simulink model "pos_8mot"  (R2021a)
settings: Solver=FixedStepDiscrete  StartTime=0.0  StopTime=inf  FixedStep=0.001  RelTol=1e-3  EnableMultiTasking=on
InitFcn:
  | load("rho_CommandCalib.mat");
  | run("importCmd.m")
model workspace (MAT data in the model file):
  positionCmd = [145.742 145.741 145.741 145.74 145.74 145.739 145.738 145.738 145.737 145.737 145.736 145.735 ... (560000 elements, 70000x8)]
  tempsTraj = [25 25 20]
values from neighbouring files (symbols this model uses):
  rho_CommandCalib = [325.033 325.033 325.033 325.033 325.033 325.033 325.033 325.033 325.033 325.033 325.033 325.033 ... (80000 elements, 10000x8)]    [rho_CommandCalib.mat]
undefined symbols (not defined in the file or in its folder): rho_CommandCircXY, rho_CommandCroixTilt, rho_CommandCroixXY, rho_CommandInclinaison, rho_CommandInclinaisonInterieure, rho_CommandPickAndPlace, rho_CommandPickAndPlaceTilt, rho_CommandPickAndPlaceVertical, rho_CommandPickAndPlaceX, rho_CommandSinusZ, rho_CommandSinusZ_decentree, rho_CommandTwist
libraries: xpcethercatlib x64, slrealtimeethercatlib x36, commutil2 x19, slrealtimeobsoletelib x7
(part 3 of 3)

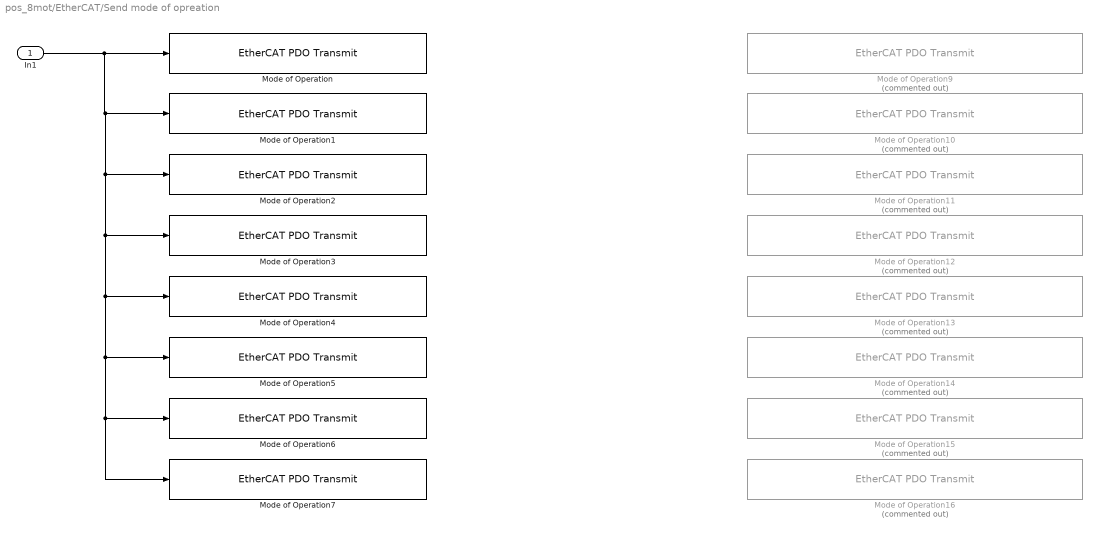
== system pos_8mot/EtherCAT/Send mode of opreation ==
  In1 : Inport
  Mode of Operation : xpcethercatlib/EtherCAT PDO Transmit   Priority=3  sig_name=Drive 1 (C1150-DS-XC-0S).Cylic Position Mode.Mode of Operation  sig_offset=744  sig_type=int8  type_size=8  sig_dim=1  device_id=0  sample_time=0.001000
      settings: SourceProductBaseCode=XP
  Mode of Operation1 : xpcethercatlib/EtherCAT PDO Transmit   Priority=3  sig_name=Drive 2 (C1150-DS-XC-0S).Cylic Position Mode.Mode of Operation  sig_offset=920  sig_type=int8  type_size=8  sig_dim=1  device_id=0  sample_time=0.001000
      settings: SourceProductBaseCode=XP
  Mode of Operation10 : xpcethercatlib/EtherCAT PDO Transmit   Priority=3  Commented=on  sig_name=Drive 2 (C1150-DS-XC-0S).Cylic Position Velocity Mode.Mode of Operation  sig_offset=936  sig_type=int8  type_size=8  sig_dim=1  device_id=0  sample_time=0.001000
      settings: SourceProductBaseCode=XP
  Mode of Operation11 : xpcethercatlib/EtherCAT PDO Transmit   Priority=3  Commented=on  sig_name=Drive 3 (C1150-DS-XC-0S).Cylic Position Velocity Mode.Mode of Operation  sig_offset=1080  sig_type=int8  type_size=8  sig_dim=1  device_id=0  sample_time=0.001000
      settings: SourceProductBaseCode=XP
  Mode of Operation12 : xpcethercatlib/EtherCAT PDO Transmit   Priority=3  Commented=on  sig_name=Drive 4 (C1150-DS-XC-0S).Cylic Position Velocity Mode.Mode of Operation  sig_offset=1224  sig_type=int8  type_size=8  sig_dim=1  device_id=0  sample_time=0.001000
      settings: SourceProductBaseCode=XP
  Mode of Operation13 : xpcethercatlib/EtherCAT PDO Transmit   Priority=3  Commented=on  sig_name=Drive 5 (C1150-DS-XC-0S).Cylic Position Velocity Mode.Mode of Operation  sig_offset=1368  sig_type=int8  type_size=8  sig_dim=1  device_id=0  sample_time=0.001000
      settings: SourceProductBaseCode=XP
  Mode of Operation14 : xpcethercatlib/EtherCAT PDO Transmit   Priority=3  Commented=on  sig_name=Drive 6 (C1150-DS-XC-0S).Cylic Position Velocity Mode.Mode of Operation  sig_offset=1512  sig_type=int8  type_size=8  sig_dim=1  device_id=0  sample_time=0.001000
      settings: SourceProductBaseCode=XP
  Mode of Operation15 : xpcethercatlib/EtherCAT PDO Transmit   Priority=3  Commented=on  sig_name=Drive 7 (C1150-DS-XC-0S).Cylic Position Velocity Mode.Mode of Operation  sig_offset=1656  sig_type=int8  type_size=8  sig_dim=1  device_id=0  sample_time=0.001000
      settings: SourceProductBaseCode=XP
  Mode of Operation16 : xpcethercatlib/EtherCAT PDO Transmit   Priority=3  Commented=on  sig_name=Drive 8 (C1150-DS-XC-0S).Cylic Position Velocity Mode.Mode of Operation  sig_offset=1800  sig_type=int8  type_size=8  sig_dim=1  device_id=0  sample_time=0.001000
      settings: SourceProductBaseCode=XP
  Mode of Operation2 : xpcethercatlib/EtherCAT PDO Transmit   Priority=3  sig_name=Drive 3 (C1150-DS-XC-0S).Cylic Position Mode.Mode of Operation  sig_offset=1080  sig_type=int8  type_size=8  sig_dim=1  device_id=0  sample_time=0.001000
      settings: SourceProductBaseCode=XP
  Mode of Operation3 : xpcethercatlib/EtherCAT PDO Transmit   Priority=3  sig_name=Drive 4 (C1150-DS-XC-0S).Cylic Position Mode.Mode of Operation  sig_offset=1240  sig_type=int8  type_size=8  sig_dim=1  device_id=0  sample_time=0.001000
      settings: SourceProductBaseCode=XP
  Mode of Operation4 : xpcethercatlib/EtherCAT PDO Transmit   Priority=3  sig_name=Drive 5 (C1150-DS-XC-0S).Cylic Position Mode.Mode of Operation  sig_offset=1400  sig_type=int8  type_size=8  sig_dim=1  device_id=0  sample_time=0.001000
      settings: SourceProductBaseCode=XP
  Mode of Operation5 : xpcethercatlib/EtherCAT PDO Transmit   Priority=3  sig_name=Drive 6 (C1150-DS-XC-0S).Cylic Position Mode.Mode of Operation  sig_offset=1560  sig_type=int8  type_size=8  sig_dim=1  device_id=0  sample_time=0.001000
      settings: SourceProductBaseCode=XP
  Mode of Operation6 : xpcethercatlib/EtherCAT PDO Transmit   Priority=3  sig_name=Drive 7 (C1150-DS-XC-0S).Cylic Position Mode.Mode of Operation  sig_offset=1720  sig_type=int8  type_size=8  sig_dim=1  device_id=0  sample_time=0.001000
      settings: SourceProductBaseCode=XP
  Mode of Operation7 : xpcethercatlib/EtherCAT PDO Transmit   Priority=3  sig_name=Drive 8 (C1150-DS-XC-0S).Cylic Position Mode.Mode of Operation  sig_offset=1880  sig_type=int8  type_size=8  sig_dim=1  device_id=0  sample_time=0.001000
      settings: SourceProductBaseCode=XP
  Mode of Operation9 : xpcethercatlib/EtherCAT PDO Transmit   Priority=3  Commented=on  sig_name=Drive 1 (C1150-DS-XC-0S).Cylic Position Velocity Mode.Mode of Operation  sig_offset=776  sig_type=int8  type_size=8  sig_dim=1  device_id=0  sample_time=0.001000
      settings: SourceProductBaseCode=XP
  wires:
  In1/1 -> Mode of Operation7/1, Mode of Operation6/1, Mode of Operation5/1, Mode of Operation4/1, Mode of Operation3/1, Mode of Operation2/1, Mode of Operation1/1, Mode of Operation/1

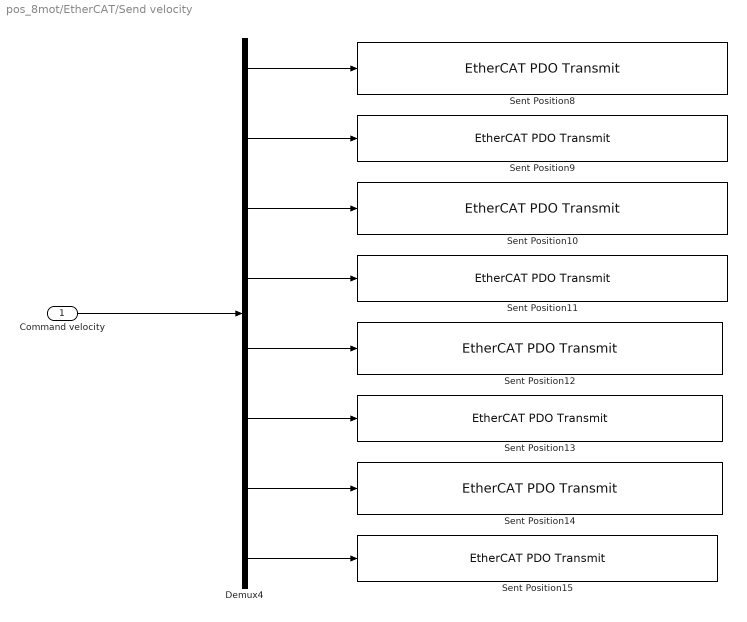
== system pos_8mot/EtherCAT/Send velocity ==
  Command velocity : Inport
  Demux4 : Demux  Outputs=8
  Sent Position10 : xpcethercatlib/EtherCAT PDO Transmit   Priority=3  sig_name=Drive 3 (C1150-DS-XC-0S).Cylic Position Velocity Mode.Target velocity  sig_offset=1048  sig_type=int32  type_size=32  sig_dim=1  device_id=0  sample_time=0.001000
      settings: SourceProductBaseCode=XP
  Sent Position11 : xpcethercatlib/EtherCAT PDO Transmit   Priority=3  sig_name=Drive 4 (C1150-DS-XC-0S).Cylic Position Velocity Mode.Target velocity  sig_offset=1192  sig_type=int32  type_size=32  sig_dim=1  device_id=0  sample_time=0.001000
      settings: SourceProductBaseCode=XP
  Sent Position12 : xpcethercatlib/EtherCAT PDO Transmit   Priority=3  sig_name=Drive 5 (C1150-DS-XC-0S).Cylic Position Velocity Mode.Target velocity  sig_offset=1336  sig_type=int32  type_size=32  sig_dim=1  device_id=0  sample_time=0.001000
      settings: SourceProductBaseCode=XP
  Sent Position13 : xpcethercatlib/EtherCAT PDO Transmit   Priority=3  sig_name=Drive 6 (C1150-DS-XC-0S).Cylic Position Velocity Mode.Target velocity  sig_offset=1480  sig_type=int32  type_size=32  sig_dim=1  device_id=0  sample_time=0.001000
      settings: SourceProductBaseCode=XP
  Sent Position14 : xpcethercatlib/EtherCAT PDO Transmit   Priority=3  sig_name=Drive 7 (C1150-DS-XC-0S).Cylic Position Velocity Mode.Target velocity  sig_offset=1624  sig_type=int32  type_size=32  sig_dim=1  device_id=0  sample_time=0.001000
      settings: SourceProductBaseCode=XP
  Sent Position15 : xpcethercatlib/EtherCAT PDO Transmit   Priority=3  sig_name=Drive 8 (C1150-DS-XC-0S).Cylic Position Velocity Mode.Target velocity  sig_offset=1768  sig_type=int32  type_size=32  sig_dim=1  device_id=0  sample_time=0.001000
      settings: SourceProductBaseCode=XP
  Sent Position8 : xpcethercatlib/EtherCAT PDO Transmit   Priority=3  sig_name=Drive 1 (C1150-DS-XC-0S).Cylic Position Velocity Mode.Target velocity  sig_offset=744  sig_type=int32  type_size=32  sig_dim=1  device_id=0  sample_time=0.001000
      settings: SourceProductBaseCode=XP
  Sent Position9 : xpcethercatlib/EtherCAT PDO Transmit   Priority=3  sig_name=Drive 2 (C1150-DS-XC-0S).Cylic Position Velocity Mode.Target velocity  sig_offset=904  sig_type=int32  type_size=32  sig_dim=1  device_id=0  sample_time=0.001000
      settings: SourceProductBaseCode=XP
  wires:
  Demux4/1 -> Sent Position8/1
  Demux4/4 -> Sent Position11/1
  Demux4/7 -> Sent Position14/1
  Demux4/2 -> Sent Position9/1
  Demux4/8 -> Sent Position15/1
  Demux4/6 -> Sent Position13/1
  Demux4/5 -> Sent Position12/1
  Demux4/3 -> Sent Position10/1
  Command velocity/1 -> Demux4/1

== matlab function pos_8mot/EtherCAT/MATLAB Function8 ==
  data: y output; u input
function y = clignote(u)


frequence_clignotement = 1; % 1 fois par seconde
frequence_solver = 1000; % Hz

mode = u(1);

reset_counter = u(2);

persistent etat;
if isempty(etat)
    etat = 0; % Éteinte
end

persistent i;
if isempty(i)
    i = 1;
elseif reset_counter == 1
    i = 1;
    etat = 0;
    mode = 0;
end



if mode == 0
    etat = 0; % Éteinte
    
elseif mode == 1
      
    etat = 1; % Allumée
    
elseif mode == 0.5 % Clignote

    if i > frequence_solver/frequence_clignotement % Fréquence de clignotement de 1 Hz
        i = 0;
        % Changement d'état
        if etat == 1
            etat = 0;
        else
            etat = 1;
        end
    end
    
else
    etat = 0; % Éteinte
end
    

i = i + 1;

if i > 60*60*24*frequence_solver % Number of increment in 1 day at frequence_solver Hz
    
    i = 1;
    
end


y = etat;

== matlab function pos_8mot/EtherCAT/MATLAB Function9 ==
  data: trajectorySelector input; target output size=[1 8]; pause input; stopAtEnd input; isCompleted output; waitForActivation input; position_from_gabarit_to_standby input; positionCmd parameter; tempsTraj parameter
function [target,isCompleted] = trajectoryManager(trajectorySelector,pause,stopAtEnd,waitForActivation,position_from_gabarit_to_standby, positionCmd, tempsTraj)

	% Constants declaration
	persistent index %index of the table trajectory
	if isempty(index)
		index = 1;
	end
	
	
	persistent flag_stopAtEnd % To stop the endless loop trajectory at the end of current trajectory
    if isempty(flag_stopAtEnd)
		flag_stopAtEnd = 0;
    end
    
    persistent numTraj
    persistent currentTime
    persistent currentIndex
    if isempty(numTraj)
        numTraj = 1;
        currentTime = tempsTraj(numTraj); %Init temps de la première trajectoire
        currentIndex = 2;
    end
	
	
	persistent pos %position of the actuator of the robot
	if isempty(pos) % Les valeurs de calibrations
		pos = [325, 323.80, 325, 325, 293.60, 293.25, 316.76, 318.94]; % 1x8 vector TO CHANGE WITH REAL CALIBRATION VALUES
	%     pos = 325; % For tests with only 1 actuator
	
	end
	
	
	
	trajectory_completed = 0; % Output variable to know if we've reach the end of a trajectory
	
	% Trajectory management
	
	
	if ~waitForActivation % If we are currently in a moving procedure
		
	
		if trajectorySelector == 1 % Trajectory from gabarit to standby
	
		   if index == length(position_from_gabarit_to_standby)
	
			   trajectory_completed = 1;
			   index = 1;
			   pos =  position_from_gabarit_to_standby(end,:);
		   else
			   if ~pause
				   index = index + 1;
			   end
			   
			   % Because of unit delay to notify that the trajectory is
			   % completed, the last command sent to actuators won't be when
			   % index = length(trajectory), but index = 1 because of the
			   % re-initialization of index when index = length(trajectory). To
			   % prevent this discontinuity in the position command, we must
			   % ensure that if the present position of actuators corresponds
			   % to the last position of trajectory vector, then we hold that
			   % position. Not optimal, but functionnal.
			   if pos ~= position_from_gabarit_to_standby(end,:)
				   
				   pos =  position_from_gabarit_to_standby(index,:);
			   else
				   
				   pos = position_from_gabarit_to_standby(end,:);
			   end
		   end
	
	
	
		elseif trajectorySelector == 2 % Trajectory from standby to gabarit
	
		   if index == length(position_from_gabarit_to_standby)
	
			   trajectory_completed = 1;
			   index = 1;
			   pos =  position_from_gabarit_to_standby(1,:);
		   else
			   if ~pause
				   index = index + 1;
			   end
			   
			   if pos ~= position_from_gabarit_to_standby(1,:)
				   
				   % Reading Trajectory_from_gabarit_to_standby backway
				   pos =  position_from_gabarit_to_standby(length(position_from_gabarit_to_standby)-index+1,:);
			   else
				   pos = position_from_gabarit_to_standby(1,:);
			   end  
		   end
	
	
	
	
	
	
	
	
		elseif trajectorySelector == 3 % Endless loop demo trajectory

			if currentIndex == currentTime * 1000
				currentIndex = 0;
                if numTraj == length(tempsTraj)     % After completing the last demo trajectory, we start again the neverending loop
                    index = 1;
                    pos =  positionCmd(end,:);
                    numTraj = 1;
                    currentIndex = 1;
                else
                    numTraj = numTraj + 1;
                end
                currentTime = tempsTraj(numTraj);
                
                if stopAtEnd
					trajectory_completed = 1;
                    index = 1;
                    numTraj = 1;
                    currentTime = tempsTraj(numTraj);
                    currentIndex = 1;
                end
			else
				if ~pause
					index = index + 1;
                    currentIndex = currentIndex + 1;
				end
				pos =  positionCmd(index,:);
			end
		else
			
			% Do nothing, stay in the current configuration
	
		end
	
	else
		
		% Holds the current configuration with persistent variable pos
		
	end
	
	
	target = pos;
	isCompleted = trajectory_completed;
	
	end

== matlab function pos_8mot/EtherCAT/Activation1/controlWord Generator ==
  data: mode output; controlword output; action input; stop input
function [mode, controlword] = fcn(action, stop)
%#codegen

persistent power
if isempty(power)
    power = 0;
end
persistent homing
if isempty(homing)
    homing = 0;
end

controlword = [0;0;1;0;0;0];
mode = 8;
if stop == 0
    if action==1 %arret
        controlword = [0;0;1;0;0;0];
        power = 0;
    elseif action==2 %homing de la position du moteur
        mode = 6;
        if power==0
            controlword = [0;1;1;1;0;0];
            power = 1;
        elseif power==1 && homing==0
            controlword = [1;1;1;1;0;0];
            homing = 1;
        elseif homing==1
            controlword = [1;1;1;1;1;0];
        end
    elseif action==3 %active la drive
        if power==0
            controlword = [0;1;1;1;0;0];
            power = 1;
        else
            controlword = [1;1;1;1;0;0];
        end
    elseif action==4 %reset fautes
        controlword = [0;1;1;1;0;1];
        power = 0;
        homing = 0;
    end
end

== matlab function pos_8mot/EtherCAT/MATLAB Function ==
  data: y output; u input
function y = clignote(u)


mode = u(1);

frequence_clignotement = 1; % 1 fois par seconde
frequence_solver = 1000; % Hz



persistent i;
if isempty(i)
    i = 1;
% elseif resetCounter == 1 % Changement d'état
%     i = 1;
end

persistent etat;
if isempty(etat)
    etat = 0; % Éteinte
end

if mode == 0
    etat = 0; % Éteinte
    
elseif mode == 1
    etat = 1; % Allumée
    
elseif mode == 0.5 % Clignote

    if i > frequence_solver/frequence_clignotement % Fréquence de clignotement de 1 Hz
        i = 0;
        % Changement d'état
        if etat == 1
            etat = 0;
        else
            etat = 1;
        end
    end
    
else
    etat = 0; % Éteinte
end
    

i = i + 1;

if i > 60*60*24*frequence_solver % Number of increment in 1 day at frequence_solver Hz
    
    i = 1;
    
end


y = etat;

== matlab function pos_8mot/EtherCAT/MATLAB Function1 ==
  data: buttonState input; isPressed output
% This function determines if a button has been pressed, in other words, if
% a rising edge followed by a falling edge has been detected.

% buttonState [0,1]

function isPressed = buttonPressed(buttonState)


buttonState = double(buttonState);

% Variable declaration

frequence_solver = 1000; % Hz

minimumPulseWidth = 0.1*frequence_solver; % Minimum allowable pulse width to accept pushed button, sec*Hz

isPressed = 0;

persistent i;
if isempty(i)
    i = 1;
end

persistent i_risingEdge;
if isempty(i_risingEdge)
    i_risingEdge = 1;
end

persistent i_fallingEdge;
if isempty(i_fallingEdge)
    i_fallingEdge = 1;
end


persistent pastState;
if isempty(pastState)
    pastState = 0;
end

persistent presentState;
if isempty(presentState)
    presentState = 0;
else
    presentState = buttonState;
end






% Rising edge detection
if pastState == 0 && presentState == 1

    i_risingEdge = i;

end

% Falling edge detection
if pastState == 1 && presentState == 0

    i_fallingEdge = i;
    
    if i_fallingEdge - i_risingEdge > minimumPulseWidth % To avoid button flickering
        
        isPressed = 1;
        
    else
        
        isPressed = 0;
        
    end

end




i = i + 1;

if i > 60*60*24*frequence_solver % Number of increments in 1 day at frequence_solver Hz
    
    i = 1;
    
end


pastState = presentState;


end

== matlab function pos_8mot/EtherCAT/MATLAB Function2 ==
  data: input input; new_state output; state input; output output
function [new_state,output] = fcn(input,state)

STATE_INIT = 0; 
STATE_WAIT_ECAT = 1; % wait ecat 8
STATE_WAIT_GABARIT_BUTTON = 2; 
STATE_CALIBRATION = 3; % set offsets for actuators
STATE_WAIT_INIT_MOVE_BUTTON = 4; 
STATE_DO_INITIAL_MOVE = 5; 
STATE_WAIT_NEW_TRAJ_BUTTON = 6; 
STATE_DO_REFERENCE_MOVE = 7; 
STATE_DO_REFERENCE_MOVE_LAST = 8; 
STATE_END = 100; 

ecat_state = input(1); 
button_1 = input(2); 
button_2 = input(3); 
button_3 = input(4); 
init_traj_end = input(5); 
ref_traj_end = input(6); 

new_state = -1; 

if state == STATE_INIT
    new_state = STATE_WAIT_ECAT; 
elseif state == STATE_WAIT_ECAT
    if ecat_state == 8
        new_state = STATE_WAIT_GABARIT_BUTTON; 
    else
        new_state = STATE_WAIT_ECAT; 
    end
elseif state == STATE_WAIT_GABARIT_BUTTON
    if button_1 == 1
        new_state = STATE_CALIBRATION; 
    else
        new_state = STATE_WAIT_GABARIT_BUTTON; 
    end
elseif state == STATE_CALIBRATION
    new_state = STATE_WAIT_INIT_MOVE_BUTTON; 
elseif state == STATE_WAIT_INIT_MOVE_BUTTON
    if button_2 == 1
        new_state = STATE_DO_INITIAL_MOVE; 
    else
        new_state = STATE_WAIT_INIT_MOVE_BUTTON; 
    end
elseif state == STATE_DO_INITIAL_MOVE
    if init_traj_end == 1
        new_state = STATE_WAIT_NEW_TRAJ_BUTTON; 
    else
        new_state = STATE_DO_INITIAL_MOVE; 
    end
elseif state == STATE_WAIT_NEW_TRAJ_BUTTON
    if button_3 == 1
        new_state = STATE_DO_REFERENCE_MOVE; 
    else
        new_state = STATE_WAIT_NEW_TRAJ_BUTTON; 
    end
elseif state == STATE_DO_REFERENCE_MOVE
    if button_1 == 1
        new_state = STATE_DO_REFERENCE_MOVE_LAST; 
    else
        new_state = STATE_DO_REFERENCE_MOVE; 
    end
elseif state == STATE_DO_REFERENCE_MOVE_LAST
    if ref_traj_end == 1
        new_state = STATE_END; 
    else
        new_state = STATE_DO_REFERENCE_MOVE_LAST; 
    end
end











output = 0; 

if state == STATE_INIT
    output = 0; 
elseif state == STATE_WAIT_ECAT
    output = 0; 
elseif state == STATE_WAIT_GABARIT_BUTTON
    output = 0; 
elseif state == STATE_CALIBRATION
    output = 0; 
elseif state == STATE_WAIT_INIT_MOVE_BUTTON
    output = 0; 
elseif state == STATE_DO_INITIAL_MOVE
    output = 1; 
end



% new_states = fcn(inputs,states); 

end

== matlab function pos_8mot/EtherCAT/MATLAB Function3 ==
  data: buttonState input; isPressed output
% This function determines if a button has been pressed, in other words, if
% a rising edge followed by a falling edge has been detected.

% buttonState [0,1]

function isPressed = buttonPressed(buttonState)


buttonState = double(buttonState);

% Variable declaration

frequence_solver = 1000; % Hz

minimumPulseWidth = 0.1*frequence_solver; % Minimum allowable pulse width to accept pushed button, sec*Hz

isPressed = 0;

persistent i;
if isempty(i)
    i = 1;
end

persistent i_risingEdge;
if isempty(i_risingEdge)
    i_risingEdge = 1;
end

persistent i_fallingEdge;
if isempty(i_fallingEdge)
    i_fallingEdge = 1;
end


persistent pastState;
if isempty(pastState)
    pastState = 0;
end

persistent presentState;
if isempty(presentState)
    presentState = 0;
else
    presentState = buttonState;
end






% Rising edge detection
if pastState == 0 && presentState == 1

    i_risingEdge = i;

end

% Falling edge detection
if pastState == 1 && presentState == 0

    i_fallingEdge = i;
    
    if i_fallingEdge - i_risingEdge > minimumPulseWidth % To avoid button flickering
        
        isPressed = 1;
        
    else
        
        isPressed = 0;
        
    end

end




i = i + 1;

if i > 60*60*24*frequence_solver % Number of increment in 1 day at frequence_solver Hz
    
    i = 1;
    
end


pastState = presentState;

% isPressed = presentState;

end

== matlab function pos_8mot/EtherCAT/MATLAB Function4 ==
  data: buttonState input; isPressed output
% This function determines if a button has been pressed, in other words, if
% a rising edge followed by a falling edge has been detected.

% buttonState [0,1]

function isPressed = buttonPressed(buttonState)


buttonState = double(buttonState);

% Variable declaration

frequence_solver = 1000; % Hz

minimumPulseWidth = 0.1*frequence_solver; % Minimum allowable pulse width to accept pushed button, sec*Hz

isPressed = 0;

persistent i;
if isempty(i)
    i = 1;
end

persistent i_risingEdge;
if isempty(i_risingEdge)
    i_risingEdge = 1;
end

persistent i_fallingEdge;
if isempty(i_fallingEdge)
    i_fallingEdge = 1;
end


persistent pastState;
if isempty(pastState)
    pastState = 0;
end

persistent presentState;
if isempty(presentState)
    presentState = 0;
else
    presentState = buttonState;
end






% Rising edge detection
if pastState == 0 && presentState == 1

    i_risingEdge = i;

end

% Falling edge detection
if pastState == 1 && presentState == 0

    i_fallingEdge = i;
    
    if i_fallingEdge - i_risingEdge > minimumPulseWidth % To avoid button flickering
        
        isPressed = 1;
        
    else
        
        isPressed = 0;
        
    end

end




i = i + 1;

if i > 60*60*24*frequence_solver % Number of increment in 1 day at frequence_solver Hz
    
    i = 1;
    
end


pastState = presentState;

% isPressed = presentState;

end

== matlab function pos_8mot/EtherCAT/MATLAB Function5 ==
  data: outputs_LED output; outputs_traj output; selectionMode output; motorPower output; inputs input; statusWordLinMot input; warnWord input size=[16, 8]; isCompleted input; new_state output; state input
function [outputs_LED,outputs_traj,selectionMode,motorPower,new_state] = stateMachine(inputs,statusWordLinMot, warnWord,isCompleted,state)

STATE_INIT = 0; 
STATE_WAIT_ECAT = 1; % wait ecat 8
STATE_WAIT_GABARIT_BUTTON = 2; % wait until the user has placed the gabarit
STATE_CALIBRATION = 3; % set offsets for actuators
STATE_WAIT_BUTTON_INIT_MOVE_TO_STANDBY = 4; 
STATE_MOVE_TO_STANDBY_FROM_GABARIT = 5; 
STATE_WAIT_TRAJECTORY_BUTTON = 6; 
STATE_ON_TRAJECTORY = 7; 
STATE_WAIT_GABARIT_BUTTON_FROM_STANDBY = 8;
STATE_MOVING_TO_GABARIT = 9;
STATE_PAUSE_TRAJECTORY = 10;
STATE_MOVE_TO_STANDBY_FROM_TRAJECTORY = 11;
STATE_PAUSE_TO_STANDBY_FROM_TRAJECTORY = 12;
STATE_PAUSE_TO_STANDBY_FROM_GABARIT = 13;
STATE_PAUSE_TO_GABARIT_FROM_STANDBY = 14;


STATE_TEMPERATURE_WARNING = 100;


button_1 = inputs(1); 
button_2 = inputs(2); 
button_3 = inputs(3);
ecat_state = inputs(4);

% fault = any(statusWordLinMot(1:8)); % Determine if any element of the array is nonzero
isHomed = all(statusWordLinMot(9:16)); % Determine if all elements of the array are nonzero

% High temperature warnings
motorHot = any(warnWord(1,:));
driveHot = any(warnWord(7,:));
regenerativeResistorHot = any(warnWord(11,:));


if ~isempty(isCompleted)
    trajectoryCompleted = isCompleted;
else
    trajectoryCompleted = 0;
end



new_state = -1; 
state_change = 0;
outputs_LED = [0;1;0;1;0;1;state_change];

trajectorySelector = 0;
pause = 0;
stopAtEnd = 0;
waitForActivation = 1;

outputs_traj = [trajectorySelector,pause,stopAtEnd,waitForActivation];


selectionMode = 1;


persistent robot_calibrated; % To assure that the robot may be calibrated only once 
if isempty(robot_calibrated)
    robot_calibrated = 0;
end

timeDelay_calibration = 3000; % ms, time delay to remain in the Calibration state

persistent counter;
if isempty(counter)
    counter = 0;
end


persistent motorPowerSupply; % Power activation in motors
if isempty(motorPowerSupply)
    motorPowerSupply = 0;
end

persistent temperatureWarning; % Warning from motor, drive or regenerative resistance hot temparature
if isempty(temperatureWarning)
    temperatureWarning = 0;
elseif motorHot || driveHot || regenerativeResistorHot
    temperatureWarning = 1;
end



% WARNING : We do not have a protection against more than one button being
% pressed at the same time.

% Initial state
if state == STATE_INIT % 0
    new_state = STATE_WAIT_ECAT;
    
% Waiting state for the operational status EtherCAT
elseif state == STATE_WAIT_ECAT % 1
    if ecat_state == 8
        new_state = STATE_WAIT_GABARIT_BUTTON; 
    else
        new_state = STATE_WAIT_ECAT; 
    end
    
    
% Waiting state for the user to place the calibration frame (gabarit)
elseif state == STATE_WAIT_GABARIT_BUTTON % 2
    if button_1 == 1 && robot_calibrated == 0
        new_state = STATE_CALIBRATION; 
        
    else
        new_state = STATE_WAIT_GABARIT_BUTTON; 
    end
    
% Calibration state. Dictates the relative position of the rods w/r to the
% stators when the platform is mechanically constrained.
elseif state == STATE_CALIBRATION % 3
    
    
    if counter < timeDelay_calibration
        
        counter = counter + 1;
        new_state = STATE_CALIBRATION;
    elseif isHomed && counter >= timeDelay_calibration
        % Produce output calibration here
        robot_calibrated = 1;
        counter = 0;
        new_state = STATE_WAIT_BUTTON_INIT_MOVE_TO_STANDBY; 
    else
        new_state = STATE_CALIBRATION;
    end
    
    
    
% Waiting state for the user to move the robot to the standby configuration, or to stop the procedure.    
elseif state == STATE_WAIT_BUTTON_INIT_MOVE_TO_STANDBY % 4
    
    if temperatureWarning
        new_state = STATE_TEMPERATURE_WARNING; 
    elseif button_2 == 1
        new_state = STATE_MOVE_TO_STANDBY_FROM_GABARIT; 
    else
        new_state = STATE_WAIT_BUTTON_INIT_MOVE_TO_STANDBY; 
    end
    
% State of the robot during a trajectory leading to the standby configuration.  
elseif state == STATE_MOVE_TO_STANDBY_FROM_GABARIT % 5
    
    % Besoin de savoir quand on est arrivé à la configuration STANDBY!!!
    if trajectoryCompleted == 1
        new_state = STATE_WAIT_TRAJECTORY_BUTTON; 
    elseif button_1 == 1
        new_state = STATE_PAUSE_TO_STANDBY_FROM_GABARIT;
    else
        new_state = STATE_MOVE_TO_STANDBY_FROM_GABARIT; 
    end

elseif state == STATE_PAUSE_TO_STANDBY_FROM_GABARIT % 13
    if button_1 == 1
        new_state = STATE_MOVE_TO_STANDBY_FROM_GABARIT;
    else
        new_state = STATE_PAUSE_TO_STANDBY_FROM_GABARIT;
    end
    
% Waiting state for the user to start the endless loop trajectory of the robot. 
elseif state == STATE_WAIT_TRAJECTORY_BUTTON % 6
    if temperatureWarning
        new_state = STATE_MOVING_TO_GABARIT;
    elseif button_3 == 1
        new_state = STATE_ON_TRAJECTORY; 
    elseif button_2 == 1
        new_state = STATE_WAIT_GABARIT_BUTTON_FROM_STANDBY; % To go back to the calibration frame
    else
        new_state = STATE_WAIT_TRAJECTORY_BUTTON; 
    end
    
% State of the robot during its endless loop trajectory.
elseif state == STATE_ON_TRAJECTORY % 7
    if temperatureWarning
        new_state = STATE_MOVE_TO_STANDBY_FROM_TRAJECTORY;
    elseif button_3 == 1
        new_state = STATE_MOVE_TO_STANDBY_FROM_TRAJECTORY; 
    elseif button_1 == 1
        new_state = STATE_PAUSE_TRAJECTORY; 
    else
        new_state = STATE_ON_TRAJECTORY; 
    end

elseif state == STATE_PAUSE_TRAJECTORY % 10
    if button_1 == 1
        new_state = STATE_ON_TRAJECTORY;
    else
        new_state = STATE_PAUSE_TRAJECTORY;
    end
    
elseif state == STATE_MOVE_TO_STANDBY_FROM_TRAJECTORY % 11
    
    if button_1 == 1
        new_state = STATE_PAUSE_TO_STANDBY_FROM_TRAJECTORY;
    elseif trajectoryCompleted == 1 
        new_state = STATE_WAIT_TRAJECTORY_BUTTON;
    else
        new_state = STATE_MOVE_TO_STANDBY_FROM_TRAJECTORY;
    end

elseif state == STATE_PAUSE_TO_STANDBY_FROM_TRAJECTORY % 12
    if button_1 == 1
        new_state = STATE_MOVE_TO_STANDBY_FROM_TRAJECTORY;
    else
        new_state = STATE_PAUSE_TO_STANDBY_FROM_TRAJECTORY;
    end
    
% Waiting state of the robot in the standby configuration for the user to
% install the calibration frame
elseif state == STATE_WAIT_GABARIT_BUTTON_FROM_STANDBY % 8    
   
    if button_2 == 1 
        new_state = STATE_MOVING_TO_GABARIT;
    else
        new_state = STATE_WAIT_GABARIT_BUTTON_FROM_STANDBY;
    end
    
% State of the robot going from the standby configuration into the
% calibration frame
elseif state == STATE_MOVING_TO_GABARIT % 9
      
    % Besoin de savoir quand on est arrivé à la configuration STANDBY!!

    if trajectoryCompleted == 1 
        new_state = STATE_WAIT_BUTTON_INIT_MOVE_TO_STANDBY; 
    elseif button_1 == 1
        new_state = STATE_PAUSE_TO_GABARIT_FROM_STANDBY;
    else
        new_state = STATE_MOVING_TO_GABARIT; 
    end

elseif state == STATE_PAUSE_TO_GABARIT_FROM_STANDBY % 14
    if button_1 == 1
        new_state = STATE_MOVING_TO_GABARIT;
    else
        new_state = STATE_PAUSE_TO_GABARIT_FROM_STANDBY;
    end
    
% Temperature warning state : we should not be able to move the robot from
% now on
elseif state == STATE_TEMPERATURE_WARNING % 100
    new_state = STATE_TEMPERATURE_WARNING;
    
end


% State change detection for blinking LED synchronization purposes
if new_state ~= state
    state_change = 1;
else
    state_change = 0;
end


% outputs_LED

% Light output format : 7x1 matrix
% 2 rows for each light (3 lights in total)
% Row #1 Light #1 : 0/0.5/1 = TurnedOff/Blinking/TurnedOn
% Row #2 Light #1 : 1/2/3 = Green/Red/Yellow
% Etc.
% Last row specifies if state has changed (to reset counters for blinking lights)


if state == STATE_WAIT_ECAT % 1
    outputs_LED = [1;2;1;2;1;2;state_change];
    
elseif state == STATE_WAIT_GABARIT_BUTTON % 2
    outputs_LED = [0.5;2;0;2;0;2;state_change]; 
    
elseif state == STATE_CALIBRATION % 3
    outputs_LED = [1;3;1;3;1;3;state_change];  
    
elseif state == STATE_WAIT_BUTTON_INIT_MOVE_TO_STANDBY % 4
    outputs_LED = [0.5;3;0;2;0;2;state_change];
    
elseif state == STATE_MOVE_TO_STANDBY_FROM_GABARIT % 5
    outputs_LED = [0.5;3;0.5;3;0.5;3;state_change];
    
elseif state == STATE_WAIT_TRAJECTORY_BUTTON % 6
    if temperatureWarning % To notify a warning for temperature was flagged
        outputs_LED = [0.5;2;0.5;2;0.5;2;state_change]; 
    else
        outputs_LED = [0.5;1;0.5;1;0.5;1;state_change];
    end
    
elseif state == STATE_ON_TRAJECTORY % 7
    outputs_LED = [1;1;1;1;1;1;state_change];
    
elseif state == STATE_WAIT_GABARIT_BUTTON_FROM_STANDBY % 8
    outputs_LED = [0.5;3;0;2;0;2;state_change];
    
elseif state == STATE_MOVING_TO_GABARIT % 9
    if temperatureWarning % To notify a warning for temperature was flagged
        outputs_LED = [0.5;2;0.5;2;0.5;2;state_change]; 
    else
        outputs_LED = [0.5;3;0.5;3;0.5;3;state_change];
    end
    
elseif state == STATE_PAUSE_TRAJECTORY % 10
    outputs_LED = [1;2;0;2;0;2;state_change];
    
elseif state == STATE_MOVE_TO_STANDBY_FROM_TRAJECTORY % 11
    if temperatureWarning % To notify a warning for temperature was flagged
        outputs_LED = [0.5;2;0.5;2;0.5;2;state_change]; 
    else
        outputs_LED = [0.5;3;0.5;3;0.5;3;state_change];
    end

elseif state == STATE_PAUSE_TO_STANDBY_FROM_TRAJECTORY % 12
    outputs_LED = [1;2;0;2;0;2;state_change];
    
elseif state == STATE_PAUSE_TO_STANDBY_FROM_GABARIT % 13
    outputs_LED = [1;2;0;2;0;2;state_change];
    
elseif state == STATE_PAUSE_TO_GABARIT_FROM_STANDBY % 14
    outputs_LED = [1;2;0;2;0;2;state_change];
    
elseif state == STATE_TEMPERATURE_WARNING % 100
    outputs_LED = [0.5;2;0.5;2;0.5;2;state_change]; 
    
end
    



% outputs_traj
% Output for starting, pausing and ending an current trajectory


if state == STATE_WAIT_ECAT % 1
    
    trajectorySelector = 0;
    pause = 0;
    stopAtEnd = 0;
    waitForActivation = 1;
    
    % OUTPUT for ''mode selection''
    selectionMode = 1;
    
    motorPowerSupply = 0;

    
elseif state == STATE_WAIT_GABARIT_BUTTON % 2
    
    trajectorySelector = 0;
    pause = 0;
    stopAtEnd = 0;
    waitForActivation = 1;
    
    % OUTPUT for ''mode selection''
    
    % WATCHOUT : Fault variable corresponds to ANY error, must not assume
    % it is only for low power supply to motors.
%     if fault % Due to low power supply to motors error
%         selectionMode = 4; % Fault reset
%     else
%         selectionMode = 1;
%     end
    
    selectionMode = 1;
    motorPowerSupply = 1;
    
elseif state == STATE_CALIBRATION % 3
    
    trajectorySelector = 0;
    pause = 0;
    stopAtEnd = 0;
    waitForActivation = 1;
    
    % OUTPUT for ''mode selection''
    selectionMode = 2;
    
    
    motorPowerSupply = 1;
    
elseif state == STATE_WAIT_BUTTON_INIT_MOVE_TO_STANDBY % 4
    
    
    trajectorySelector = 0;
    pause = 0;
    stopAtEnd = 0;
    waitForActivation = 1;
    
    
    % OUTPUT for ''mode selection''
    selectionMode = 3;
    
    motorPowerSupply = 1;
    
elseif state == STATE_MOVE_TO_STANDBY_FROM_GABARIT % 5
       
    trajectorySelector = 1;
    pause = 0;
    stopAtEnd = 0;
    waitForActivation = 0;
    
    
    % OUTPUT for ''mode selection''
    selectionMode = 3;
    
    motorPowerSupply = 1;
    
elseif state == STATE_WAIT_TRAJECTORY_BUTTON % 6
    
    
    trajectorySelector = 0;
    pause = 0;
    stopAtEnd = 0;
    waitForActivation = 1;
    
    % OUTPUT for ''mode selection''
    selectionMode = 3;
    
    motorPowerSupply = 1;
    
elseif state == STATE_ON_TRAJECTORY % 7
    
    trajectorySelector = 3;
    pause = 0;
    stopAtEnd = 0;
    waitForActivation = 0;
    
    
    % OUTPUT for ''mode selection''
    selectionMode = 3;
    
    motorPowerSupply = 1;
    
elseif state == STATE_WAIT_GABARIT_BUTTON_FROM_STANDBY % 8
    
    trajectorySelector = 0;
    pause = 0;
    stopAtEnd = 0;
    waitForActivation = 1;
    
    
    % OUTPUT for ''mode selection''
    selectionMode = 3;
    
    motorPowerSupply = 1;
    
elseif state == STATE_MOVING_TO_GABARIT % 9
    
    trajectorySelector = 2;
    pause = 0;
    stopAtEnd = 0;
    waitForActivation = 0;
    
    
    % OUTPUT for ''mode selection''
    selectionMode = 3;
    
    motorPowerSupply = 1;
    
elseif state == STATE_PAUSE_TRAJECTORY % 10
    
    trajectorySelector = 3;
    pause = 1;
    stopAtEnd = 0;
    waitForActivation = 0;
    
    
    % OUTPUT for ''mode selection''
    selectionMode = 3;
    
    motorPowerSupply = 1;
    
elseif state == STATE_MOVE_TO_STANDBY_FROM_TRAJECTORY % 11
    
    trajectorySelector = 3;
    pause = 0;
    stopAtEnd = 1;
    waitForActivation = 0;
    
    
    % OUTPUT for ''mode selection''
    selectionMode = 3;
    
    motorPowerSupply = 1;

elseif state == STATE_PAUSE_TO_STANDBY_FROM_TRAJECTORY % 12
    
    trajectorySelector = 3;
    pause = 1;
    stopAtEnd = 1;
    waitForActivation = 0;
    
    
    
    % OUTPUT for ''mode selection''
    selectionMode = 3;
    
    motorPowerSupply = 1;
    
elseif state == STATE_PAUSE_TO_STANDBY_FROM_GABARIT % 13
    
    
    trajectorySelector = 1;
    pause = 1;
    stopAtEnd = 0;
    waitForActivation = 0;
    
    
    % OUTPUT for ''mode selection''
    selectionMode = 3;
    
    motorPowerSupply = 1;
    
elseif state == STATE_PAUSE_TO_GABARIT_FROM_STANDBY % 14
    
    trajectorySelector = 2;
    pause = 1;
    stopAtEnd = 0;
    waitForActivation = 0;
    
    
    % OUTPUT for ''mode selection''
    selectionMode = 3;
    
    motorPowerSupply = 1;
    
elseif state == STATE_TEMPERATURE_WARNING % 100
    
    
    trajectorySelector = 0;
    pause = 0;
    stopAtEnd = 0;
    waitForActivation = 1;
    
    
    % OUTPUT for ''mode selection''
    selectionMode = 1;
    
    motorPowerSupply = 0;
    
end


outputs_traj = [trajectorySelector,pause,stopAtEnd,waitForActivation];

motorPower = motorPowerSupply;


end

== matlab function pos_8mot/EtherCAT/MATLAB Function6 ==
  data: y output; u input
function y = clignote(u)


frequence_clignotement = 1; % 1 fois par seconde
frequence_solver = 1000; % Hz

mode = u(1);

reset_counter = u(2);

persistent etat;
if isempty(etat)
    etat = 0; % Éteinte
end

persistent i;
if isempty(i)
    i = 1;
elseif reset_counter == 1
    i = 1;
    etat = 0;
    mode = 0;
end



if mode == 0
    etat = 0; % Éteinte
    
elseif mode == 1
      
    etat = 1; % Allumée
    
elseif mode == 0.5 % Clignote

    if i > frequence_solver/frequence_clignotement % Fréquence de clignotement de 1 Hz
        i = 0;
        % Changement d'état
        if etat == 1
            etat = 0;
        else
            etat = 1;
        end
    end
    
else
    etat = 0; % Éteinte
end
    

i = i + 1;

if i > 60*60*24*frequence_solver % Number of increment in 1 day at frequence_solver Hz
    
    i = 1;
    
end


y = etat;

== matlab function pos_8mot/EtherCAT/MATLAB Function7 ==
  data: y output; u input
function y = clignote(u)


frequence_clignotement = 1; % 1 fois par seconde
frequence_solver = 1000; % Hz

mode = u(1);

reset_counter = u(2);

persistent etat;
if isempty(etat)
    etat = 0; % Éteinte
end

persistent i;
if isempty(i)
    i = 1;
elseif reset_counter == 1
    i = 1;
    etat = 0;
    mode = 0;
end



if mode == 0
    etat = 0; % Éteinte
    
elseif mode == 1
      
    etat = 1; % Allumée
    
elseif mode == 0.5 % Clignote

    if i > frequence_solver/frequence_clignotement % Fréquence de clignotement de 1 Hz
        i = 0;
        % Changement d'état
        if etat == 1
            etat = 0;
        else
            etat = 1;
        end
    end
    
else
    etat = 0; % Éteinte
end
    

i = i + 1;

if i > 60*60*24*frequence_solver % Number of increment in 1 day at frequence_solver Hz
    
    i = 1;
    
end


y = etat;
